simulink model "torqueDistribution"  (R2019b)
settings: Solver=VariableStepAuto  StartTime=0.0  StopTime=10.0  RelTol=1e-3
values from neighbouring files (symbols this model uses):
  Rd = 0.2    [runTorqueVectoringScript.m]
  tr = 1.1    [runTorqueVectoringScript.m]
settings Model: Creator=mha483  LastModifiedBy=mha483

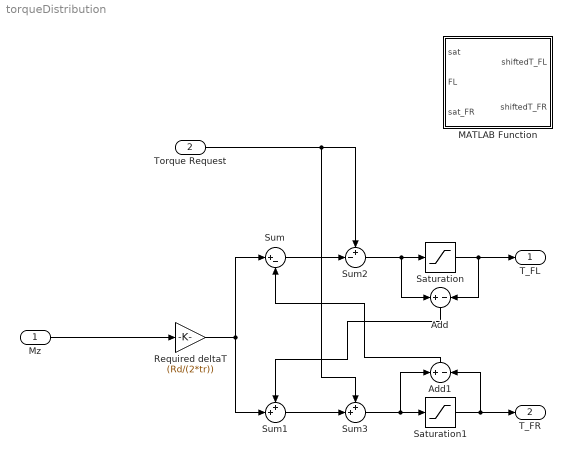
== system torqueDistribution ==
  Mz : Inport
  Torque Request : Inport  Port=2
  Add : Sum  Inputs=+|-
  Add1 : Sum  Inputs=+|-
  MATLAB Function : MATLAB Function  TreatAsAtomicUnit=on
  Required deltaT : Gain  Gain=(Rd/(2*tr))
  Saturation : Saturate  UpperLimit=1000  LowerLimit=-1000
  Saturation1 : Saturate  UpperLimit=1000  LowerLimit=-1000
  Sum : Sum  Inputs=|+-
  Sum1 : Sum  Inputs=++|
  Sum2 : Sum  Inputs=+-|
  Sum3 : Sum  Inputs=++|
  T_FL : Outport
  T_FR : Outport  Port=2
  wires:
  Mz/1 -> Required deltaT/1
  Torque Request/1 -> Sum2/1, Sum3/1
  Sum/1 -> Sum2/2
  Sum1/1 -> Sum3/2
  Sum3/1 -> Saturation1/1, Add1/1
  Saturation/1 -> T_FL/1, Add/2
  Add1/1 -> Sum/2
  Required deltaT/1 -> Sum/1, Sum1/2
  Saturation1/1 -> T_FR/1, Add1/2
  Sum2/1 -> Saturation/1, Add/1
  Add/1 -> Sum1/1

== matlab function torqueDistribution/MATLAB Function ==
  data: sat input; shiftedT_FL output; FL input; sat_FR input; shiftedT_FR output
function [shiftedT_FL,shiftedT_FR] = fcn(sat,FL,sat_FR)

y = u;
